simulink model "MidSideProcessor_ProgSim_Start"  (R2026a)
settings: Solver=FixedStepDiscrete  StopTime=inf
libraries: MidSideLibrary_Solution x2, dspsnks4 x1, dspvision x1
settings Model: Creator=Adam  LastModifiedBy=skerber
settings DebuggingCC: AlgebraicLoopMsg=error  SingleTaskRateTransMsg=error

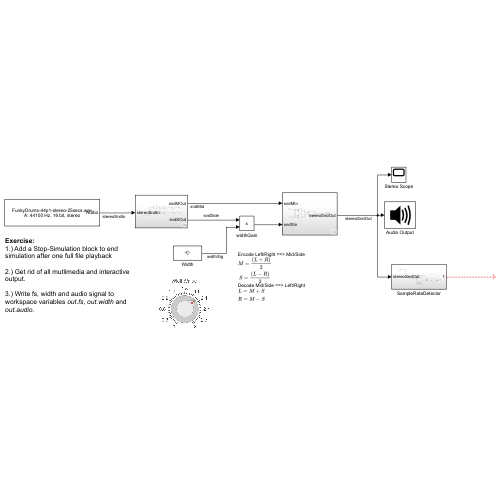
[thumbnail: Simulink's stored preview of the top-level diagram]
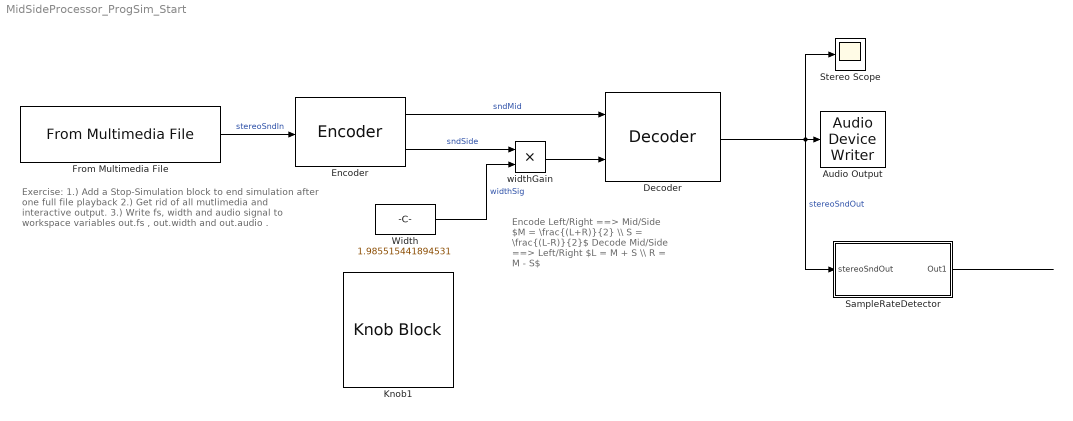
== system MidSideProcessor_ProgSim_Start ==
  note: Exercise:
      | 1.) Add a Stop-Simulation block to end simulation after one full file playback
      |
      | 2.) Get rid of all mutlimedia and interactive output.
      |
      | 3.) Write fs, width and audio signal to workspace variables out.fs , out.width and out.audio .
  note: Encode Left/Right ==> Mid/Side
      | $M = \frac{(L+R)}{2} \\ S = \frac{(L-R)}{2}$
      | Decode Mid/Side ==> Left/Right
      | $L = M + S \\ R = M - S$
  Audio Output : dspsnks4/Audio Device Writer  Driver=DirectSound  Device=Default  InheritSampleRate=on  SampleRate=44100  BitDepth=16-bit integer  BufferSize=4096  NumBuffers=10  DefaultOutputChannelMapping=on  OutputChannelMapping=1:2  OutputNumUnderrunSamples=off  DriverIdx=1  DeviceWarnFlag=''
  Decoder : MidSideLibrary_Solution/Decoder  SystemSampleTime=-1  VariantActivationTime=update diagram  EmptyChoice=off  PassThrough=off  PassThroughVariantControl=(default)  EmptyChoiceVariantControl=(default)  AllowFlexibleInterface=on  Latency=0  AutoFrameSizeCalculation=off
  Encoder : MidSideLibrary_Solution/Encoder  SystemSampleTime=-1  VariantActivationTime=update diagram  EmptyChoice=off  PassThrough=off  PassThroughVariantControl=(default)  EmptyChoiceVariantControl=(default)  AllowFlexibleInterface=on  Latency=0  AutoFrameSizeCalculation=off
  From Multimedia File : dspvision/From Multimedia File  inputFilename=FunkyDrums-44p1-stereo-25secs.wav  readRange=[1 Inf]  loop=on  numPlays=1  outputStreams=Audio only  videoDataType=single  audioDataType=double  inheritSampleTime=on  userDefinedSampleTime=1/30  noAudioOutput=off  isIntensityVideo=off  fourcc=RGB  colorVideoFormat=Separate color signals  outputEOF=off  dataOrg=Column-major  audioFrameSize=1024  computeAudioFrameSize=off  outSamplingMode=Sample based
  Knob1 : KnobBlock  ScaleMax=3
  SampleRateDetector : Subsystem
  Stereo Scope : Scope
      settings: TimeUnits=Metric (based on Time Span)  ActiveDisplayYMinimum=-0.94246292114257812  ActiveDisplayYMaximum=1.0020027160644531  YLabel=Amplitude
  Width : Constant  Value=1.985515441894531
  widthGain : Product
  wires:
  Width/1 -> widthGain/2  "widthSig"
  From Multimedia File/1 -> Encoder/1  "stereoSndIn"
  Decoder/1 -> SampleRateDetector/1(stereoSndOut), Stereo Scope/1, Audio Output/1  "stereoSndOut"
  Encoder/1 -> Decoder/1  "sndMid"
  widthGain/1 -> Decoder/2
  Encoder/2 -> widthGain/1  "sndSide"
  SampleRateDetector/1(Out1) -> ?

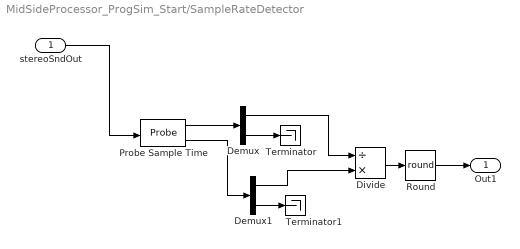
== system MidSideProcessor_ProgSim_Start/SampleRateDetector ==
  stereoSndOut : Inport
  Demux : Demux  Outputs=2
  Demux1 : Demux  Outputs=2
  Divide : Product  Inputs=/*
  Probe Sample Time : Probe  ProbeWidth=off  ProbeComplexSignal=off  ProbeSignalDimensions=on
  Round : Rounding  Operator=round
  Terminator : Terminator
  Terminator1 : Terminator
  Out1 : Outport
  wires:
  Demux/2 -> Terminator/1
  Divide/1 -> Round/1
  Demux1/2 -> Terminator1/1
  Probe Sample Time/2 -> Demux1/1
  Probe Sample Time/1 -> Demux/1
  Demux/1 -> Divide/1
  Round/1 -> Out1/1
  Demux1/1 -> Divide/2
  stereoSndOut/1 -> Probe Sample Time/1
